simulink model "model02"  (Simulink 7.9)
settings: Solver=ode45  StartTime=0.0  StopTime=10.0  RelTol=1e-3
values from neighbouring files (symbols this model uses):
  Kp = 1    [M2_ol.m]
  T = 1/125    (= 0.008)    [M2_ol.m]
undefined symbols (not defined in the file or in its folder): initE
settings Model: Creator=ex16  LastModifiedBy=ex16

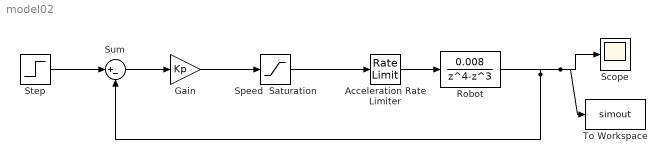
== system model02 ==
  Acceleration Rate Limiter : RateLimiter  RisingSlewLimit=15  FallingSlewLimit=-15  SampleTimeMode=inherited
  Gain : Gain  Gain=Kp  SampleTime=T
  Robot : DiscreteTransferFcn  Numerator=[0.008]  Denominator=[1 -1 0 0 0]  SampleTime=T
  Scope : Scope
  Speed  Saturation : Saturate  UpperLimit=3.2  LowerLimit=-3.2  SampleTime=T
  Step : Step  Time=0  After=initE  SampleTime=T
  Sum : Sum  Inputs=|+-
  To Workspace : ToWorkspace  VariableName=simout  SampleTime=-1  SaveFormat=Structure With Time
  wires:
  Gain/1 -> Speed  Saturation/1
  Sum/1 -> Gain/1
  Robot/1 -> Sum/2, To Workspace/1, Scope/1
  Step/1 -> Sum/1
  Speed  Saturation/1 -> Acceleration Rate Limiter/1
  Acceleration Rate Limiter/1 -> Robot/1
